simulink model "constant_gain_variable_Q"  (Simulink 7.4)
settings: Solver=ode45  StartTime=0.0  StopTime=inf  RelTol=1e-4
PreLoadFcn:
  | f2=100e6;f1=10e6;Av=200;
StartFcn:
  | tic;
StopFcn:
  | t=toc
undefined symbols (not defined in the file or in its folder): Fs, magnitude
libraries: powerlib x12, dspindex x6, dspsigops x3, dsparch4 x3, dspbuff3 x2, dspxfrm3 x2, dsparch3 x2, simulink x2, dspmtrx3 x1, dspsnks4 x1
settings Model: Creator=Owner  LastModifiedBy=Dick
settings DataIOCC: SignalLoggingName=sigsOut
settings OptimizationCC: InlineInvariantSignals=on  InitFltsAndDblsToZero=on
settings DebuggingCC: SaveWithParameterizedLinksMsg=none  SignalResolutionControl=TryResolveAllWithWarning  SolverPrmCheckMsg=none  MultiTaskDSMMsg=warning  MultiTaskCondExecSysMsg=none  StrictBusMsg=None
settings HardwareCC: TargetUnknown=on
settings RTWCC: IncludeERTFirstTime=on
settings GRTTargetCC: TargetFcnLib=ansi_tfl_tmw.mat

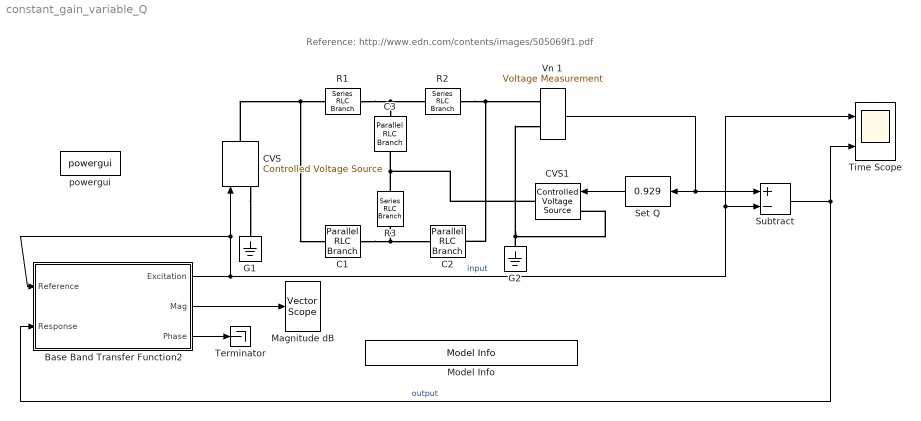
== system constant_gain_variable_Q ==
  note: Reference: http://www.edn.com/contents/images/505069f1.pdf
  Base Band Transfer Function2 : Subsystem  Description=Spectrum Analyzer  mask{BW=10e3, NFFT=1024, Avg_fac=2}
      mask prompts: BW "Bandwidth"; NFFT "FFT Length (power of 2)"; Avg_fac "Averaging Factor (>=1)"
  C1 : powerlib/Elements/Parallel RLC Branch  DialogController=POWERSYS.PowerSysDialog  PhysicalDomain=powersysdomain  SubClassName=unknown  LeftPortType=p1  RightPortType=p1  LConnTagsString=a  RConnTagsString=__new0  BranchType=C  Resistance=1.0  Inductance=1.0  SetiL0=off  InitialCurrent=0  Capacitance=0.01e-6  Setx0=off  InitialVoltage=0  Measurements=None
  C2 : powerlib/Elements/Parallel RLC Branch  DialogController=POWERSYS.PowerSysDialog  PhysicalDomain=powersysdomain  SubClassName=unknown  LeftPortType=p1  RightPortType=p1  LConnTagsString=a  RConnTagsString=__new0  BranchType=C  Resistance=1.0  Inductance=1.0  SetiL0=off  InitialCurrent=0  Capacitance=0.01e-6  Setx0=off  InitialVoltage=0  Measurements=None
  C3 : powerlib/Elements/Parallel RLC Branch  DialogController=POWERSYS.PowerSysDialog  PhysicalDomain=powersysdomain  SubClassName=unknown  LeftPortType=p1  RightPortType=p1  LConnTagsString=a  RConnTagsString=__new0  BranchType=C  Resistance=1.0  Inductance=1.0  SetiL0=off  InitialCurrent=0  Capacitance=2*0.01e-6  Setx0=off  InitialVoltage=0  Measurements=None
  CVS : powerlib/Electrical Sources/Controlled Voltage Source  Description=source block  DialogController=POWERSYS.PowerSysDialog  SystemSampleTime=-1  Initialize=off  Source_Type=AC  Amplitude=0  Phase=0  Frequency=0  Measurements=None
      settings: AttributesFormatString=\n
  CVS1 : powerlib/Electrical Sources/Controlled Voltage Source  Description=source block  DialogController=POWERSYS.PowerSysDialog  SystemSampleTime=-1  Initialize=off  Source_Type=AC  Amplitude=0  Phase=0  Frequency=0  Measurements=None
      settings: AttributesFormatString=\n
  G1 : powerlib/Elements/Ground  DialogController=POWERSYS.PowerSysDialog  PhysicalDomain=powersysdomain  SubClassName=unknown  LeftPortType=p1  RightPortType=p1  LConnTagsString=a
  G2 : powerlib/Elements/Ground  DialogController=POWERSYS.PowerSysDialog  PhysicalDomain=powersysdomain  SubClassName=unknown  LeftPortType=p1  RightPortType=p1  LConnTagsString=a
  Magnitude dB : dspsnks4/Vector Scope  DialogController=dspdialog.VectorScope  DialogControllerArgs=DataTag5  ScopeProperties=on  Domain=Frequency  HorizSpan=1  DisplayProperties=off  AxisGrid=on  Memory=off  FrameNumber=on  AxisLegend=off  AxisZoom=off  OpenScopeAtSimStart=on  OpenScopeImmediately=off  FigPos=[15 321 372 236]  AxisProperties=off  XUnits=Hertz  XRange=[0...Fs/2]  InheritXIncr=on  XIncr=2*Fs  XLabel=Time  XLimit=Auto  XMin=0  XMax=1  XStart=0  YUnits=dB  YLabel=dB  LineProperties=off  LineColors=[1 0 0]|[1 0 0]  XAxisParamsVer=6.9
      settings: YMin=-100  YMax=10
  Model Info : simulink/Model-Wide Utilities/Model Info  SystemSampleTime=-1  InitialBlockCM=None  BlockCM=None  Frame=on  DisplayStringWithTags=Copywrite 2005-2010 The MathWorks, Inc.  HorizontalTextAlignment=Center  LeftAlignmentValue=0.5  SourceBlockDiagram=constant_gain_variable_Q  TagMaxNumber=20
  "R1 " : powerlib/Elements/Series RLC Branch  DialogController=POWERSYS.PowerSysDialog  PhysicalDomain=powersysdomain  SubClassName=unknown  LeftPortType=p1  RightPortType=p1  LConnTagsString=__new0  RConnTagsString=__new0  BranchType=R  Resistance=1e4  Inductance=1.0  SetiL0=off  InitialCurrent=0  Capacitance=1.0  Setx0=off  InitialVoltage=0  Measurements=None
  R2 : powerlib/Elements/Series RLC Branch  DialogController=POWERSYS.PowerSysDialog  PhysicalDomain=powersysdomain  SubClassName=unknown  LeftPortType=p1  RightPortType=p1  LConnTagsString=__new0  RConnTagsString=__new0  BranchType=R  Resistance=1e4  Inductance=1.0  SetiL0=off  InitialCurrent=0  Capacitance=1.0  Setx0=off  InitialVoltage=0  Measurements=None
  R3 : powerlib/Elements/Series RLC Branch  DialogController=POWERSYS.PowerSysDialog  PhysicalDomain=powersysdomain  SubClassName=unknown  LeftPortType=p1  RightPortType=p1  LConnTagsString=__new0  RConnTagsString=__new0  BranchType=R  Resistance=1e4/2  Inductance=1.0  SetiL0=off  InitialCurrent=0  Capacitance=1.0  Setx0=off  InitialVoltage=0  Measurements=None
  Set Q : simulink/Math Operations/Slider Gain  SystemSampleTime=-1  low=0.7  gain=0.929  high=1
  Subtract : Sum  Inputs=+-  OutDataType=sfix(16)  OutScaling=2^-10
  Terminator : Terminator
  Time Scope : Scope  NumInputPorts=2
      settings: TimeRange=0.06  YMin=-2~-0.4  YMax=2~0.4  DataFormat=Structure
  Vn 1 : powerlib/Measurements/Voltage Measurement  Tag=PoWeRsYsTeMmEaSuReMeNt  DialogController=POWERSYS.PowerSysDialog  SystemSampleTime=-1  PhasorSimulation=off  OutputType=Magnitude  PSBequivalent=0
  powergui : powerlib/powergui  SystemSampleTime=-1  SimulationMode=Continuous  SampleTime=0  frequency=60  SPID=off  DisableSnubberDevices=off  DisableRonSwitches=off  DisableVfSwitches=off  SwTol=0  Interpol=off  frequencyindice=0  echomessages=off  HookPort=off  DisplayEquations=off  FunctionMessages=off  EnableUseOfTLC=off  x0status=blocks  RestoreLinks=warning  Frange=[0:2:500]  Ylog=off  Xlog=on  ShowGrid=off  save=off  variable=ZData  ZoomFFT=on  StartTime=0.0  cycles=1  DisplayStyle=1  fundamental=60  FreqAxis=off  MaxFrequency=1000  frequencyindicesteady=1  RmsSteady=1  display=off  Ts=0  methode=off
  wires:
  Subtract/1 -> Time Scope/2, Base Band Transfer Function2/2(Response)  "output"
  Base Band Transfer Function2/1(Excitation) -> CVS/1, Base Band Transfer Function2/1("Reference "), Subtract/2, Time Scope/1  "input"
  Vn 1/1 -> Subtract/1, Set Q/1
  Set Q/1 -> CVS1/1
  Base Band Transfer Function2/2(Mag) -> Magnitude dB/1
  Base Band Transfer Function2/3(Phase) -> Terminator/1
  connections:
  CVS/LConn1 -- G1/LConn1
  CVS/RConn1 -- "R1 "/RConn1 -- C1/LConn1
  "R1 "/LConn1 -- R2/RConn1 -- C3/LConn1
  C1/RConn1 -- C2/LConn1 -- R3/LConn1
  R2/LConn1 -- C2/RConn1 -- Vn 1/LConn1
  G2/LConn1 -- Vn 1/LConn2 -- CVS1/LConn1
  R3/RConn1 -- C3/RConn1 -- CVS1/RConn1

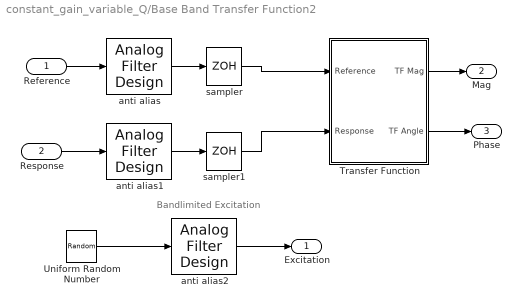
== system constant_gain_variable_Q/Base Band Transfer Function2 ==
  note: Bandlimited Excitation
  "Reference " : Inport  OutDataType=sfix(16)  OutScaling=2^0
  Response : Inport  Port=2  OutDataType=sfix(16)  OutScaling=2^0
  "Transfer Function " : Subsystem  mask{NFFT=NFFT, Navg=Avg_fac, pcnt=100/1.28, unwrap_flag=on}
      mask prompts: NFFT "FFT length (power of 2):"; Navg "Spectral Averaging Factor (>=1):"; pcnt "Percentage of  Alias Free Data  (<=100)"; unwrap_flag "Unwrap Phase"
      mask Display: disp('Transfer Function \n Estimation (v2.0) ')
  Uniform Random Number : UniformRandomNumber  SampleTime=1/(2.56*BW)
  anti alias : dsparch4/Analog Filter Design  method=Elliptic  filttype=Lowpass  N=8  Wlo=BW*2*pi  Whi=80  Rp=2  Rs=100
  anti alias1 : dsparch4/Analog Filter Design  method=Elliptic  filttype=Lowpass  N=8  Wlo=BW*2*pi  Whi=80  Rp=2  Rs=100
  anti alias2 : dsparch4/Analog Filter Design  method=Elliptic  filttype=Lowpass  N=8  Wlo=BW*2*pi  Whi=80  Rp=2  Rs=100
  sampler : ZeroOrderHold  SampleTime=1/(2.56*BW)
  sampler1 : ZeroOrderHold  SampleTime=1/(2.56*BW)
  Excitation : Outport  OutDataType=sfix(16)  OutScaling=2^0
  Mag : Outport  Port=2  OutDataType=sfix(16)  OutScaling=2^0
  Phase : Outport  Port=3  OutDataType=sfix(16)  OutScaling=2^0
  wires:
  "Transfer Function "/2(TF Angle) -> Phase/1
  "Transfer Function "/1(TF Mag) -> Mag/1
  sampler1/1 -> "Transfer Function "/2(Response)
  sampler/1 -> "Transfer Function "/1(Reference)
  anti alias2/1 -> Excitation/1
  Uniform Random Number/1 -> anti alias2/1
  Response/1 -> anti alias1/1
  anti alias1/1 -> sampler1/1
  "Reference "/1 -> anti alias/1
  anti alias/1 -> sampler/1

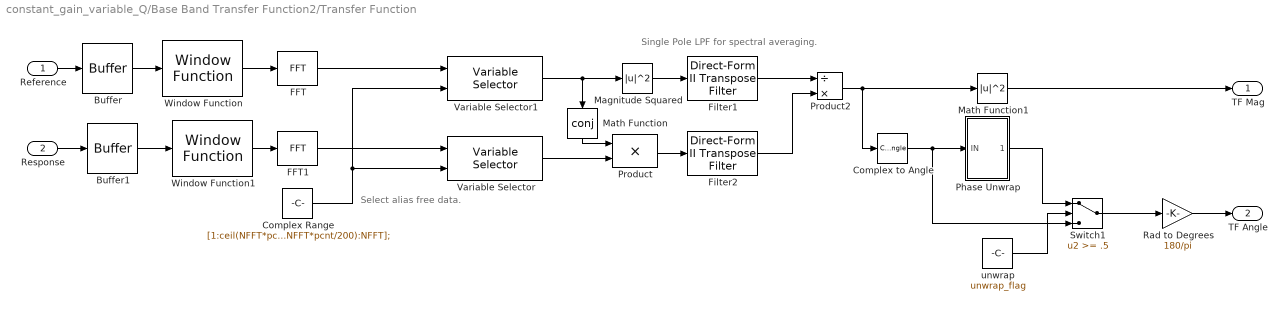
== system constant_gain_variable_Q/Base Band Transfer Function2/Transfer Function  ==
  note: Select alias free data.
  note: Single Pole LPF for spectral averaging.
  Reference : Inport  OutDataType=sfix(16)  OutScaling=2^0
  Response : Inport  Port=2  OutDataType=sfix(16)  OutScaling=2^0
  Buffer : dspbuff3/Buffer  N=NFFT  V=0  ic=0
  Buffer1 : dspbuff3/Buffer  N=NFFT  V=0  ic=0
  Complex Range : Constant  Value=[1:ceil(NFFT*pcnt/200),ceil(1+NFFT-NFFT*pcnt/200):NFFT];  OutDataType=sfix(16)  OutScaling=2^0
  Complex to Angle : ComplexToMagnitudeAngle  Output=Angle
  FFT : dspxfrm3/FFT  DialogController=dspDDGCreate  DialogControllerArgs=DataTag0  CompMethod=Table lookup  TableOpt=NEW  TableOptActive=Speed  BitRevOrder=off  InheritFFTLength=on  FFTLength=64  SkipNorm=on  firstCoeffMode=Specify word length  firstCoeffWordLength=16  firstCoeffFracLength=15  roundingMode=Floor  overflowMode=off
  FFT1 : dspxfrm3/FFT  DialogController=dspDDGCreate  DialogControllerArgs=DataTag1  CompMethod=Table lookup  TableOpt=NEW  TableOptActive=Speed  BitRevOrder=off  InheritFFTLength=on  FFTLength=64  SkipNorm=on  firstCoeffMode=User-defined  firstCoeffWordLength=16  firstCoeffFracLength=15  roundingMode=Floor  overflowMode=off
  Filter1 : dsparch3/Direct-Form II Transpose Filter  num=1  den=[Navg -(Navg-1)]  ic=eps
  Filter2 : dsparch3/Direct-Form II Transpose Filter  num=1  den=[Navg -(Navg-1)]  ic=eps
  Magnitude Squared : Math  Operator=magnitude^2  OutDataType=sfix(16)  OutScaling=2^0  SaturateOnIntegerOverflow=on
  Math Function : Math  Operator=conj  OutDataType=sfix(16)  OutScaling=2^0  SaturateOnIntegerOverflow=on
  Math Function1 : Math  Operator=magnitude^2  OutDataType=sfix(16)  OutScaling=2^0  SaturateOnIntegerOverflow=on
  Phase Unwrap : Subsystem
  Product : Product  OutDataType=sfix(16)  OutScaling=2^0  SaturateOnIntegerOverflow=on  InputSameDT=on  OutDataTypeStr=Inherit: Same as first input
  Product2 : Product  Inputs=/*  OutDataType=sfix(16)  OutScaling=2^0  SaturateOnIntegerOverflow=on  InputSameDT=on  OutDataTypeStr=Inherit: Same as first input
  Rad to Degrees : Gain  Gain=180/pi  ParameterDataType=sfix(16)  ParameterScaling=2^0  OutDataType=sfix(16)  OutScaling=2^0
  Switch1 : Switch  Threshold=.5
  Variable Selector : dspindex/Variable Selector  NumInputs=1  rowsOrCols=Rows  IdxMode=Variable  Elements=[1 3]  ZerOneIdxMode=One-based  errmode=Clip Index  FillMode=on  FillValues=0
  Variable Selector1 : dspindex/Variable Selector  NumInputs=1  rowsOrCols=Rows  IdxMode=Variable  Elements=[1 3]  ZerOneIdxMode=One-based  errmode=Clip Index  FillMode=on  FillValues=0
  Window Function : dspsigops/Window Function  DialogController=dspDDGCreate  DialogControllerArgs=DataTag3  winmode=Apply window to input  wintype=Hann  sampmode=Continuous  samptime=1  N=64  Rs=50  beta=10  winsamp=Periodic  UserWindow=hamming  OptParams=off  UserParams={'symmetric'}  dataType=double  isSigned=on  wordLen=16  udDataType=sfix(16)  fracBitsMode=Best precision  numFracBits=15  roundingMode=Floor  overflowMode=off  numSidelobes=4  sidelobeLevel=-30
  Window Function1 : dspsigops/Window Function  DialogController=dspDDGCreate  DialogControllerArgs=DataTag4  winmode=Apply window to input  wintype=Hann  sampmode=Continuous  samptime=1  N=64  Rs=50  beta=10  winsamp=Periodic  UserWindow=hamming  OptParams=off  UserParams={'symmetric'}  dataType=double  isSigned=on  wordLen=16  udDataType=sfix(16)  fracBitsMode=Best precision  numFracBits=15  roundingMode=Floor  overflowMode=off  numSidelobes=4  sidelobeLevel=-30
  unwrap : Constant  Value=unwrap_flag  OutDataType=sfix(16)  OutScaling=2^0
  TF Mag : Outport  OutDataType=sfix(16)  OutScaling=2^0
  TF Angle : Outport  Port=2  OutDataType=sfix(16)  OutScaling=2^0
  wires:
  Phase Unwrap/1(Out1) -> Switch1/1
  unwrap/1 -> Switch1/2
  Switch1/1 -> Rad to Degrees/1
  Variable Selector1/1 -> Math Function/1, Magnitude Squared/1
  Variable Selector/1 -> Product/2
  Product2/1 -> Math Function1/1, Complex to Angle/1
  Buffer1/1 -> Window Function1/1
  Buffer/1 -> Window Function/1
  Filter2/1 -> Product2/2
  Filter1/1 -> Product2/1
  Window Function1/1 -> FFT1/1
  Window Function/1 -> FFT/1
  Math Function1/1 -> TF Mag/1
  FFT/1 -> Variable Selector1/1
  Magnitude Squared/1 -> Filter1/1
  Math Function/1 -> Product/1
  FFT1/1 -> Variable Selector/1
  Product/1 -> Filter2/1
  Reference/1 -> Buffer/1
  Response/1 -> Buffer1/1
  Rad to Degrees/1 -> TF Angle/1
  Complex to Angle/1 -> Phase Unwrap/1(IN), Switch1/3
  Complex Range/1 -> Variable Selector1/2, Variable Selector/2

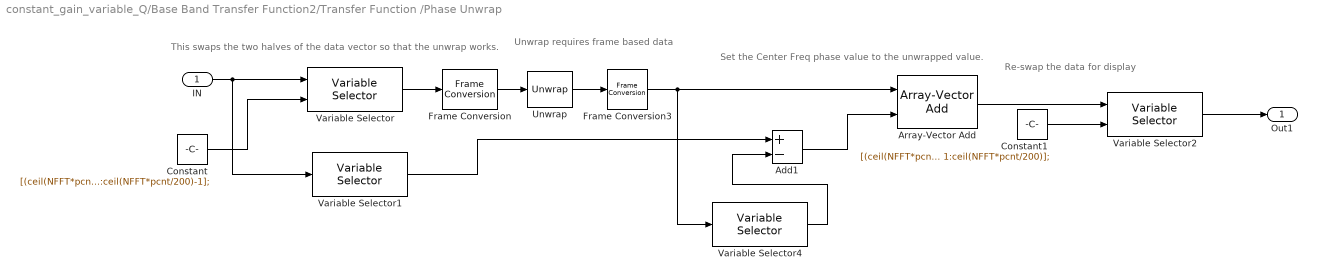
== system constant_gain_variable_Q/Base Band Transfer Function2/Transfer Function /Phase Unwrap ==
  note: Unwrap requires frame based data
  note: Re-swap the data for display
  note: Set the Center Freq phase value to the unwrapped value.
  note: This swaps the two halves of the data vector
      | so that the unwrap works.
  IN : Inport  OutDataType=sfix(16)  OutScaling=2^0
  Add1 : Sum  Inputs=+-  OutDataType=sfix(16)  OutScaling=2^-10
  Array-Vector Add : dspmtrx3/Array-Vector Add  DialogController=dspDDGCreate  DialogControllerArgs=DataTag2  Dimension=2  V_Source=Input port  V_VectFromMask=[0.5 0.25]  firstCoeffDataTypeStr=Inherit: Same word length as input  firstCoeffLastDataTypeStr=Inherit: Same word length as input  firstCoeffMin=[]  firstCoeffMax=[]  outputDataTypeStr=Inherit: Same as accumulator  outputLastDataTypeStr=Inherit: Same as accumulator  outputMin=[]  outputMax=[]  roundingMode=Floor  overflowMode=off
  Constant : Constant  Value=[(ceil(NFFT*pcnt/200)):ceil(NFFT*pcnt/100) 1:ceil(NFFT*pcnt/200)-1];  OutDataType=sfix(16)  OutScaling=2^0
  Constant1 : Constant  Value=[(ceil(NFFT*pcnt/200)+1):ceil(NFFT*pcnt/100) 1:ceil(NFFT*pcnt/200)];  OutDataType=sfix(16)  OutScaling=2^0
  Frame Conversion : FrameConversion
  Frame Conversion3 : FrameConversion  OutFrame=Sample-based
  Unwrap : dspsigops/Unwrap  running=on  tol=pi
  Variable Selector : dspindex/Variable Selector  NumInputs=1  rowsOrCols=Rows  IdxMode=Variable  Elements=[1 3]  ZerOneIdxMode=One-based  errmode=Clip Index  FillMode=on  FillValues=0
  Variable Selector1 : dspindex/Variable Selector  NumInputs=1  rowsOrCols=Rows  IdxMode=Fixed  Elements=[1]  ZerOneIdxMode=One-based  errmode=Clip Index  FillMode=on  FillValues=0
  Variable Selector2 : dspindex/Variable Selector  NumInputs=1  rowsOrCols=Rows  IdxMode=Variable  Elements=[1 3]  ZerOneIdxMode=One-based  errmode=Clip Index  FillMode=on  FillValues=0
  Variable Selector4 : dspindex/Variable Selector  NumInputs=1  rowsOrCols=Rows  IdxMode=Fixed  Elements=length([(ceil(NFFT*pcnt/200)+1):ceil(NFFT*pcnt/100) 1:ceil(NFFT*pcnt/200)] )/2+1  ZerOneIdxMode=One-based  errmode=Clip Index  FillMode=on  FillValues=0
  Out1 : Outport  OutDataType=sfix(16)  OutScaling=2^0
  wires:
  Array-Vector Add/1 -> Variable Selector2/1
  Add1/1 -> Array-Vector Add/2
  Frame Conversion3/1 -> Array-Vector Add/1, Variable Selector4/1
  Constant1/1 -> Variable Selector2/2
  Variable Selector4/1 -> Add1/2
  Unwrap/1 -> Frame Conversion3/1
  Variable Selector1/1 -> Add1/1
  Variable Selector/1 -> Frame Conversion/1
  Constant/1 -> Variable Selector/2
  IN/1 -> Variable Selector1/1, Variable Selector/1
  Variable Selector2/1 -> Out1/1
  Frame Conversion/1 -> Unwrap/1
